simulink model "MPC_Simulink_RotPen"  (R2021b)
settings: Solver=VariableStepAuto  StartTime=0.0  StopTime=1000  RelTol=1e-3
values from neighbouring files (symbols this model uses):
  A = [0 0 1 0;      0 0 0 1;      0 A_132 A_133 A_134;      0 A_142 A_143 A_144]    [PendulumParams.m]
  B = kt * B/Rm    [PendulumParams.m]
  C = [1 0 0 0]    [PendulumParams.m]
  D = [0]    [PendulumParams.m]
undefined symbols (not defined in the file or in its folder): Continuous, Time
libraries: ctrlSharedLib x1, mpclib x1
settings Model: Creator=oliverschamp  LastModifiedBy=oliverschamp

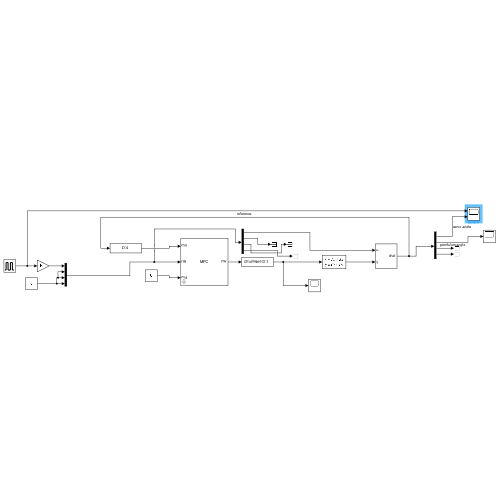
[thumbnail: Simulink's stored preview of the top-level diagram]
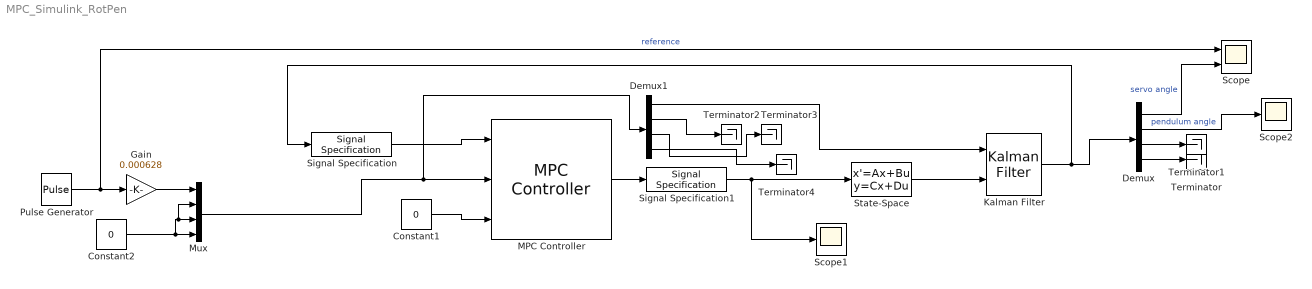
== system MPC_Simulink_RotPen ==
  Constant1 : Constant  Value=0
  Constant2 : Constant  Value=0
  Demux : Demux
  Demux1 : Demux
  Gain : Gain  Gain=0.000628
  Kalman Filter : ctrlSharedLib/Kalman Filter  TimeDomain=Continuous-Time  UseCurrentEstimator=on  ModelSource=LTI State-Space Variable  ModelSourceVariable=sys1  A=0.95  B=1  C=1  D=0  NumberOfStates=1  NumberOfInputs=1  NumberOfOutputs=1  InitialEstimateSource=Dialog  X0=[0 10 0 0]  P0=10  UseK=off  UseGH=off  NumberOfProcessNoiseInputs=1  G=1  TimeInvariantG=on  H=0  TimeInvariantH=on  Q=0.05  TimeInvariantQ=on  R=1  TimeInvariantR=on  N=0  TimeInvariantN=on  AddInputPort=on  AddEnablePort=off  OutputEstimatedY=off  OutputP=off  Ts=-1
  MPC Controller : mpclib/MPC Controller  SCDEnableBlockLinearizationSpecification=on  mpcobj=mpc1  is_multiple=0  enable_value=0  return_u0=off  updateMPCinCallerWorkspace=on  md_inport=on  mv_inport=off  uref_inport=off  return_cost=off  return_mvseq=off  return_qpstatus=off  return_xseq=off  return_state=off  return_ovseq=off  state_inport=off  umin_inport=off  umax_inport=off  ymin_inport=off  ymax_inport=off  cc_inport=off  ywt_inport=off  uwt_inport=off  duwt_inport=off  rhoeps_inport=off  pm_inport=off  MaximumP=10  HorizonChoice=FixedHorizon  n_ts=0.1  n_p=11  n_mv=1  n_md=1  n_ud=0  n_mo=4  n_uo=0  BlockDataType=double  SampleTimeInherited=off  switch_inport=off
  Mux : Mux
  Pulse Generator : DiscretePulseGenerator  PulseType=Time based  Amplitude=90  Period=600  PulseWidth=50
  Scope : Scope  NumInputPorts=2
  Scope1 : Scope
  Scope2 : Scope
  Signal Specification : SignalSpecification  Dimensions=4
  Signal Specification1 : SignalSpecification  OutDataTypeStr=double  Dimensions=1
  State-Space : StateSpace  A=A  B=B  C=C  D=D  InitialCondition=[0 10 0 0]
  Terminator{,1..4} (5 alike) : Terminator
  wires:
  Signal Specification/1 -> MPC Controller/1
  Signal Specification1/1 -> State-Space/1, Scope1/1
  MPC Controller/1 -> Signal Specification1/1
  Kalman Filter/1 -> Signal Specification/1, Demux/1
  Constant1/1 -> MPC Controller/3
  State-Space/1 -> Kalman Filter/2
  Demux/2 -> Scope2/1  "pendulum angle"
  Mux/1 -> Demux1/1, MPC Controller/2
  Demux/3 -> Terminator1/1
  Demux/4 -> Terminator/1
  Demux/1 -> Scope/2  "servo angle"
  Constant2/1 -> Mux/2, Mux/3, Mux/4
  Pulse Generator/1 -> Gain/1, Scope/1  "reference"
  Demux1/1 -> Kalman Filter/1
  Demux1/2 -> Terminator2/1
  Demux1/3 -> Terminator3/1
  Demux1/4 -> Terminator4/1
  Gain/1 -> Mux/1
